simulink model "testQueueStageModel"  (R2026a)
settings: Solver=VariableStepAuto
values from neighbouring files (symbols this model uses):
  TestCapacity = 200    [testQueueStage.m]
settings Model: Creator=aarav  LastModifiedBy=aarav

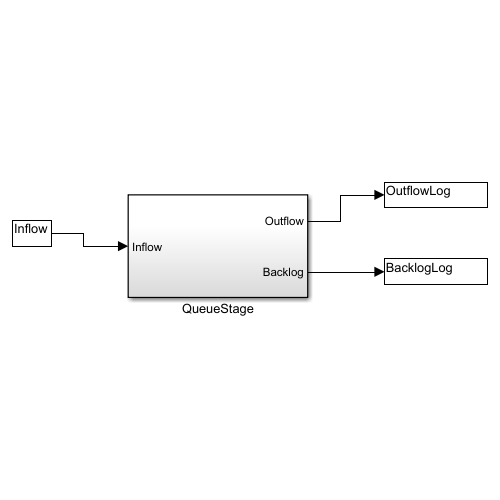
[thumbnail: Simulink's stored preview of the top-level diagram]
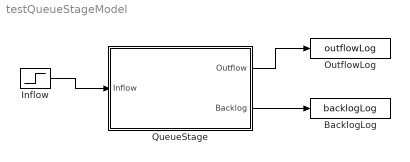
== system testQueueStageModel ==
  BacklogLog : ToWorkspace  VariableName=backlogLog  SaveFormat=Structure With Time  SampleTime=-1
  Inflow : Step  Time=0  InitialValue=100  FinalValue=100  SampleTime=0
  OutflowLog : ToWorkspace  VariableName=outflowLog  SaveFormat=Structure With Time  SampleTime=-1
  QueueStage : Subsystem
  wires:
  Inflow/1 -> QueueStage/1(Inflow)
  QueueStage/1(Outflow) -> OutflowLog/1
  QueueStage/2(Backlog) -> BacklogLog/1

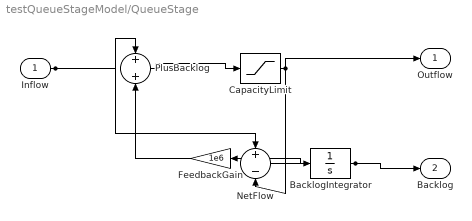
== system testQueueStageModel/QueueStage ==
  Inflow : Inport
  BacklogIntegrator : Integrator  LimitOutput=on  LowerSaturationLimit=0
  CapacityLimit : Saturate  UpperLimit=TestCapacity  LowerLimit=0
  FeedbackGain : Gain  Gain=1e6
  NetFlow : Sum  Inputs=+-
  PlusBacklog : Sum
  Outflow : Outport
  Backlog : Outport  Port=2
  wires:
  ? -> ?
  Inflow/1 -> PlusBacklog/1, NetFlow/1
  PlusBacklog/1 -> CapacityLimit/1
  CapacityLimit/1 -> Outflow/1, NetFlow/2
  NetFlow/1 -> BacklogIntegrator/1
  BacklogIntegrator/1 -> Backlog/1, FeedbackGain/1
  FeedbackGain/1 -> PlusBacklog/2
